simulink model "obserwator"  (R2014b)
settings: Solver=ode45  StartTime=0.0  StopTime=30  RelTol=1e-3
values from neighbouring files (symbols this model uses):
  T = 0.5    [zadanie1STP.m]
settings Model: Creator=KonradSob  LastModifiedBy=KonradSob

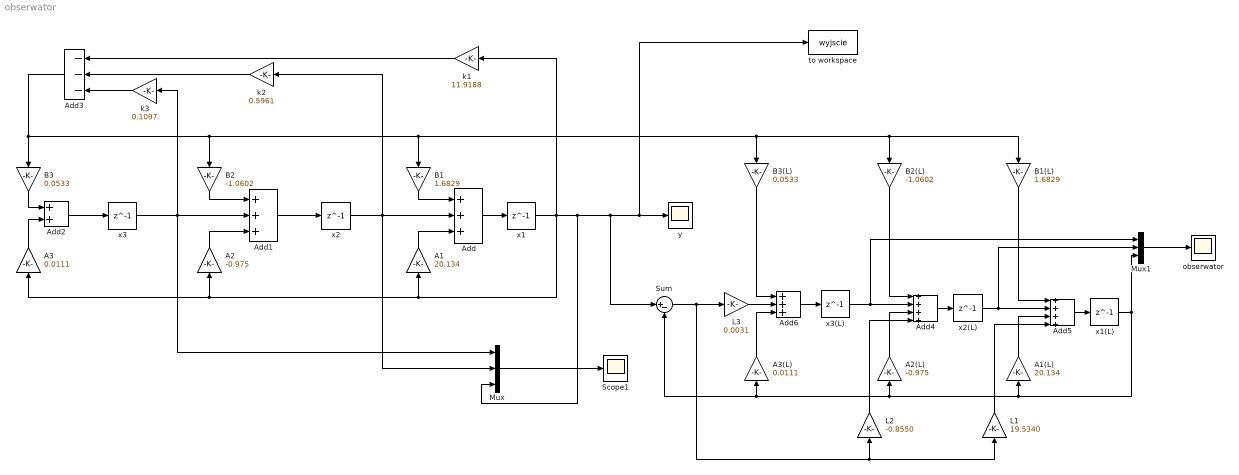
== system obserwator ==
  A1 : Gain  Gain=20.134
  A1(L) : Gain  Gain=20.134
  A2 : Gain  Gain=-0.975
  A2(L) : Gain  Gain=-0.975
  A3 : Gain  Gain=0.0111
  A3(L) : Gain  Gain=0.0111
  Add : Sum  Inputs=+++
  Add1 : Sum  Inputs=+++
  Add2 : Sum
  Add3 : Sum  Inputs=---
  Add4 : Sum  Inputs=++++
  Add5 : Sum  Inputs=++++
  Add6 : Sum  Inputs=+++
  B1 : Gain  Gain=1.6829
  B1(L) : Gain  Gain=1.6829
  B2 : Gain  Gain=-1.0602
  B2(L) : Gain  Gain=-1.0602
  B3 : Gain  Gain=0.0533
  B3(L) : Gain  Gain=0.0533
  L1 : Gain  Gain=19.5340
  L2 : Gain  Gain=-0.8550
  L3 : Gain  Gain=0.0031
  Mux : Mux  Inputs=3
  Mux1 : Mux  Inputs=3
  Scope1 : Scope
  Sum : Sum  Inputs=|+-
  k1 : Gain  Gain=11.9188
  k2 : Gain  Gain=0.5961
  k3 : Gain  Gain=0.1097
  obserwator : Scope
      settings: YMin=-1  YMax=1  SaveName=ScopeData2
  "to workspace " : ToWorkspace  VariableName=wyjscie  SaveFormat=Timeseries  SampleTime=-1
  x1 : Delay  DelayLength=1  InitialCondition=5  SampleTime=T
  "x1(L) " : Delay  DelayLength=1  InitialCondition=0  SampleTime=0.5
  x2 : Delay  DelayLength=1  InitialCondition=-1  SampleTime=T
  "x2(L) " : Delay  DelayLength=1  InitialCondition=0  SampleTime=0.5
  x3 : Delay  DelayLength=1  InitialCondition=3  SampleTime=T
  x3(L) : Delay  DelayLength=1  InitialCondition=0  SampleTime=0.5
  y : Scope
  wires:
  x1/1 -> A3/1, A2/1, A1/1, Sum/1, "to workspace "/1, y/1, Mux/3, k1/1
  x2/1 -> Mux/2, Add/2, k2/1
  Add/1 -> x1/1
  Add2/1 -> x3/1
  Add1/1 -> x2/1
  x3/1 -> Mux/1, Add1/2, k3/1
  k3/1 -> Add3/3
  k1/1 -> Add3/1
  B2/1 -> Add1/1
  Mux/1 -> Scope1/1
  A3/1 -> Add2/2
  k2/1 -> Add3/2
  B1/1 -> Add/1
  A1/1 -> Add/3
  A2/1 -> Add1/3
  B3/1 -> Add2/1
  Add3/1 -> B2/1, B3(L)/1, B2(L)/1, B1(L)/1, B1/1, B3/1
  Add5/1 -> "x1(L) "/1
  B1(L)/1 -> Add5/1
  "x2(L) "/1 -> Mux1/2, Add5/2
  "x1(L) "/1 -> Mux1/3, A2(L)/1, Sum/2, A3(L)/1, A1(L)/1
  Add4/1 -> "x2(L) "/1
  B2(L)/1 -> Add4/1
  x3(L)/1 -> Mux1/1, Add4/2
  Add6/1 -> x3(L)/1
  B3(L)/1 -> Add6/1
  A3(L)/1 -> Add6/3
  Sum/1 -> L1/1, L2/1, L3/1
  L3/1 -> Add6/2
  L2/1 -> Add4/4
  L1/1 -> Add5/4
  A2(L)/1 -> Add4/3
  A1(L)/1 -> Add5/3
  Mux1/1 -> obserwator/1
